simulink subsystem "subsistema_electromagnetico"  (R2023b)
settings: Solver=VariableStepAuto  StartTime=0.0  StopTime=10.0  RelTol=1e-3
values from neighbouring files (symbols this model uses):
  lambda_m = 0.016    [constantes.m]
  Ld = 6.6e-3    (= 0.0066)    [constantes.m]
  Lls = 0.8e-3    (= 0.0008)    [constantes.m]
  Lq = 5.8e-3    (= 0.0058)    [constantes.m]
  P_p = 3    [constantes.m]
settings Model: Creator=nahue  LastModifiedBy=nahue

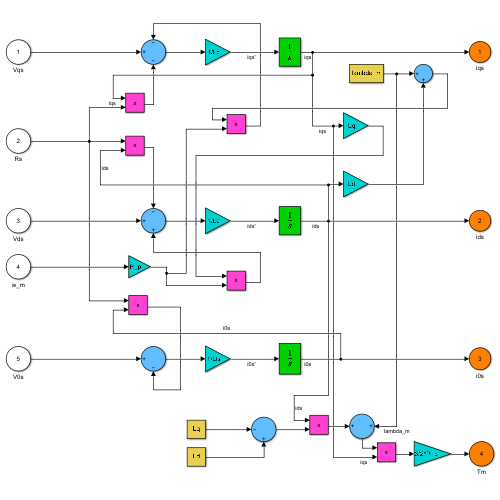
[thumbnail: Simulink's stored preview of the top-level diagram]
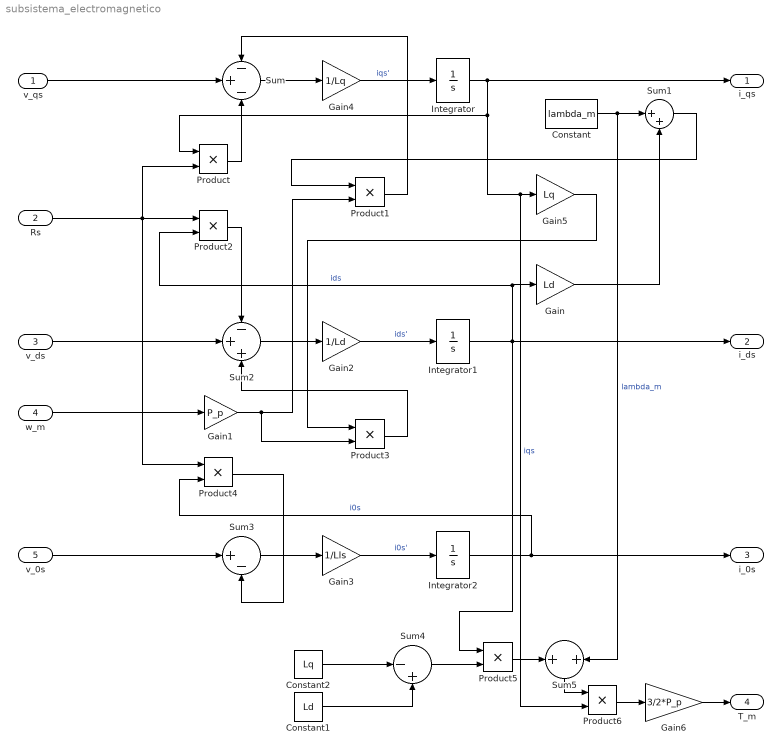
== system subsistema_electromagnetico ==
  v_qs : Inport
  Rs : Inport  Port=2
  v_ds : Inport  Port=3
  w_m : Inport  Port=4
  v_0s : Inport  Port=5
  Constant : Constant  Value=lambda_m
  Constant1 : Constant  Value=Ld
  Constant2 : Constant  Value=Lq
  Gain : Gain  Gain=Ld
  Gain1 : Gain  Gain=P_p
  Gain2 : Gain  Gain=1/Ld
  Gain3 : Gain  Gain=1/Lls
  Gain4 : Gain  Gain=1/Lq
  Gain5 : Gain  Gain=Lq
  Gain6 : Gain  Gain=3/2*P_p
  Integrator : Integrator
  Integrator1 : Integrator
  Integrator2 : Integrator
  Product{,1..6} (7 alike) : Product
  Sum : Sum  Inputs=-+-
  Sum1 : Sum  Inputs=|++
  Sum2 : Sum  Inputs=-++
  Sum3 : Sum  Inputs=|+-
  Sum4 : Sum  Inputs=|-+
  Sum5 : Sum
  i_qs : Outport
  i_ds : Outport  Port=2
  i_0s : Outport  Port=3
  T_m : Outport  Port=4
  wires:
  Rs/1 -> Product4/1, Product2/1, Product/2
  Product/1 -> Sum/3
  w_m/1 -> Gain1/1
  Gain1/1 -> Product3/2, Product1/2
  Gain/1 -> Sum1/2
  Constant/1 -> Sum5/2, Sum1/1  "lambda_m"
  Sum1/1 -> Product1/1
  Product1/1 -> Sum/1
  Sum/1 -> Gain4/1
  Gain4/1 -> Integrator/1  "iqs'"
  Integrator/1 -> Product6/2, Gain5/1, Product/1, i_qs/1  "iqs"
  Gain5/1 -> Product3/1
  v_ds/1 -> Sum2/2
  v_qs/1 -> Sum/2
  Product2/1 -> Sum2/1
  Product3/1 -> Sum2/3
  Sum2/1 -> Gain2/1
  Gain2/1 -> Integrator1/1  "ids'"
  Integrator1/1 -> Product5/1, i_ds/1, Product2/2, Gain/1  "ids"
  v_0s/1 -> Sum3/1
  Product4/1 -> Sum3/2
  Sum3/1 -> Gain3/1
  Gain3/1 -> Integrator2/1  "i0s'"
  Integrator2/1 -> i_0s/1, Product4/2  "i0s"
  Sum4/1 -> Product5/2
  Constant2/1 -> Sum4/1
  Constant1/1 -> Sum4/2
  Sum5/1 -> Product6/1
  Product6/1 -> Gain6/1
  Gain6/1 -> T_m/1
  Product5/1 -> Sum5/1
